simulink model "quadcopter_pd_test"  (R2015b)
settings: Solver=VariableStepAuto  StartTime=0.0  StopTime=20  RelTol=1e-3
undefined symbols (not defined in the file or in its folder): sigbuilder_block
libraries: vrlib x2
settings Model: Creator=Daniel  LastModifiedBy=Daniel

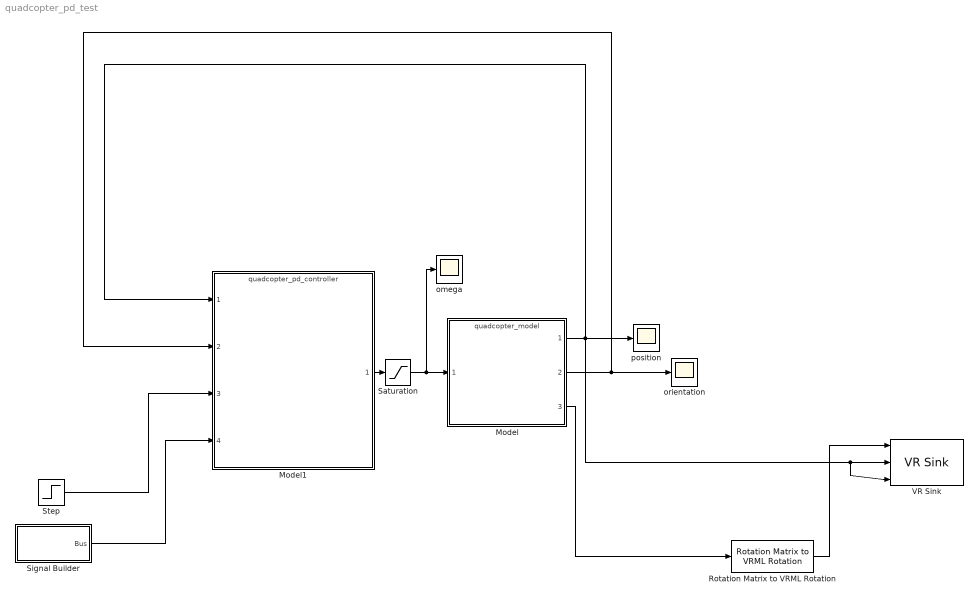
== system quadcopter_pd_test ==
  Model : ModelReference  ModelNameDialog=quadcopter_model.mdl  SimulationMode=Normal  ModelReferenceVersion=1.106  CopyOfModelName=quadcopter_model.mdl
  Model1 : ModelReference  ModelNameDialog=quadcopter_pd_controller.mdl  SimulationMode=Normal  ModelReferenceVersion=1.59  CopyOfModelName=quadcopter_pd_controller.mdl
  Rotation Matrix to VRML Rotation : vrlib/Utilities/Rotation Matrix to VRML Rotation  maxzero=1e-12
  Saturation : Saturate  UpperLimit=1000  LowerLimit=0
  Signal Builder : Subsystem  Tag=STV Subsys  LoadFcn=sigbuilder_block('load');  StartFcn=sigbuilder_block('start');  StopFcn=sigbuilder_block('stop');  ClipboardFcn=sigbuilder_block('clipboard');  mask(Sigbuilder block){}
      mask help: Simulink:masks:SigbuilderBlock_MD
      mask init:
      | if ~strcmp(get_param(bdroot(gcbh),'SimulationStatus'),'stopped') tuvar = sigbuilder_block('maskInit'); end
      settings: CopyFcn=sigbuilder_block('copy');  DeleteFcn=sigbuilder_block('delete');  ModelCloseFcn=sigbuilder_block('modelClose');  PreSaveFcn=sigbuilder_block('preSave');  PauseFcn=sigbuilder_block('pause');  ContinueFcn=sigbuilder_block('continue');  NameChangeFcn=sigbuilder_block('namechange');  OpenFcn=sigbuilder_block('open',[405 198 550.5 399.75 ]);  CloseFcn=sigbuilder_block('close');
      mask Display: plot(0, 0, 100, 100,[2, 2, 32, 32, 2], [68, 8, 8, 68, 68],[32, 2], [38, 38], [32, 19, 2],[53, 60, 44], [32, 17, 17, 2],[16, 16, 31, 31]);txt = getActiveGroup(gcbh);text(2, 100, txt,'verticalAlignment', 'top');
  Step : Step  Time=12  Before=[0 0 0]'  After=[0 0 5]'  SampleTime=0
  VR Sink : vrlib/VR Sink  InstantiateOnLoad=on  SampleTime=0.1  ViewEnable=on  RemoteChange=off  RemoteView=off  FieldsWritten=copter.rotation.4.1.1.double#copter.translation.3.1.1.double#vp.translation.3.1.1.double  WorldFileName=copter_world.wrl  WorldDescription=quadcopter_world  AutoView=on  VideoDimensions=[]  AllowVariableSize=off  FigureProperties="{'Position', 'Name', 'Viewpoint', 'CameraBound', 'CameraDirection', 'CameraPosition', 'CameraUpVector', 'ZoomFactor', 'Antialiasing', 'Headlight', 'Lighting', 'NavPanel', 'Sound', 'StatusBar', 'Stereo3D', 'Stereo3DCameraOffset', 'Stereo3DHIT', 'ToolBar', 'Textures', 'Transparency', 'Triad', 'Wireframe', 'NavZones', 'NavMode', 'NavSpeed', 'CaptureFileFormat', 'CaptureFileName', 'Record2DCompressMethod', 'Record2DCompressQuality', 'Record2D', 'Record2DFileName', 'Record2DFPS'; [5.0000000000000000e+00   9.2000000000000000e+01   5.7600000000000000e+02   3.8000000000000000e+02], 'quadcopter_world', 'viewpoint', 'on', [0.0000000000000000e+00   0.0000000000000000e+00  -1.0000000000000000e+00], [0.0000000000000000e+00   0.0000000000000000e+00   0.0000000000000000e+00], [0.0000000000000000e+00   1.0000000000000000e+00   0.0000000000000000e+00], [1.0000000000000000e+00], 'on', 'on', 'on', 'halfbar', 'on', 'on', 'off', [1.0000000149011612e-01], [0.0000000000000000e+00], 'on', 'on', 'on', 'none', 'off', 'off', 'fly', 'normal', 'tif', '%f_anim_%n.tif', 'auto', [7.5000000000000000e+01], 'off', '%f_anim_%n.avi', 'auto'}"
  "omega " : Scope
  orientation : Scope
  position : Scope
  wires:
  Model/2 -> Model1/2, orientation/1
  Model/1 -> Model1/1, VR Sink/3, VR Sink/2, position/1
  Rotation Matrix to VRML Rotation/1 -> VR Sink/1
  Signal Builder/1(Bus) -> Model1/4
  Step/1 -> Model1/3
  Model1/1 -> Saturation/1
  Saturation/1 -> Model/1, "omega "/1
  Model/3 -> Rotation Matrix to VRML Rotation/1

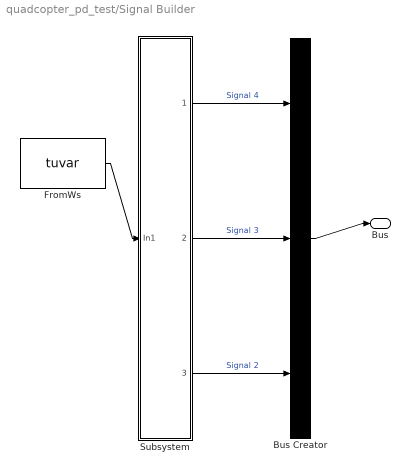
== system quadcopter_pd_test/Signal Builder ==
  Bus Creator : BusCreator  Tag=Bus Creator  Inputs=3
  FromWs : FromWorkspace  Tag=STV FromWs  VariableName=tuvar  SampleTime=0
      SigBuilderData=|
      | common.afterFinalStr = 'Extrapolate'
      | common.sampleTime = 0
      | dataSet.timeRange = [0 10]
      | dataSet.name = 'Group 1'
      | sbobj.Groups.Name = 'Group 1'
      | sbobj.Groups.Signals(1).Name = 'Signal 4'
      | sbobj.Groups.Signals(1).XData = [0 7.02 7.02 9.54 9.54 10]
      | sbobj.Groups.Signals(1).YData = [0 0 0.27 0.27 0 0]
      | sbobj.Groups.Signals(2).Name = 'Signal 3'
      | sbobj.Groups.Signals(2).XData = [0 2.6 2.6 5.08 5.08 10]
      | sbobj.Groups.Signals(2).YData = [0 0 0.22 0.22 0 0]
      | sbobj.Groups.Signals(3).Name = 'Signal 2'
      | sbobj.Groups.Signals(3).XData = [0 8.58 8.58 10]
      | sbobj.Groups.Signals(3).YData = [0 0.02 0.77 0.79]
  Subsystem : Subsystem
  Bus : Outport
  wires:
  FromWs/1 -> Subsystem/1(In1)
  Bus Creator/1 -> Bus/1
  Subsystem/1(Signal 4) -> Bus Creator/1  "Signal 4"
  Subsystem/2(Signal 3) -> Bus Creator/2  "Signal 3"
  Subsystem/3(Signal 2) -> Bus Creator/3  "Signal 2"

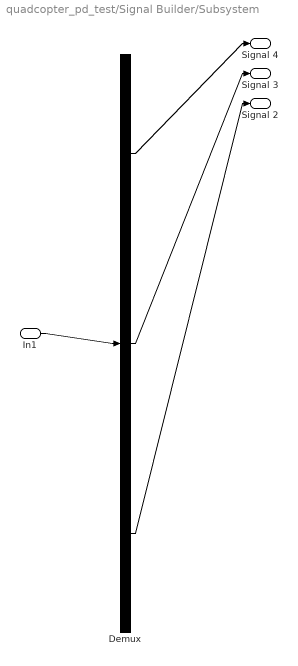
== system quadcopter_pd_test/Signal Builder/Subsystem ==
  In1 : Inport
  Demux : Demux  Tag=STV Demux  Outputs=3
  Signal 4 : Outport  Tag=STV Outport
  Signal 3 : Outport  Tag=STV Outport  Port=2
  Signal 2 : Outport  Tag=STV Outport  Port=3
  wires:
  In1/1 -> Demux/1
  Demux/1 -> Signal 4/1
  Demux/2 -> Signal 3/1
  Demux/3 -> Signal 2/1
